simulink model "Simulacao"  (R2015a)
settings: Solver=ode45  StartTime=0.0  StopTime=25  RelTol=1e-3
undefined symbols (not defined in the file): K, Kd, Ki, Kp, T, teta
settings Model: Creator=Alunos  LastModifiedBy=Miguel Gameiro

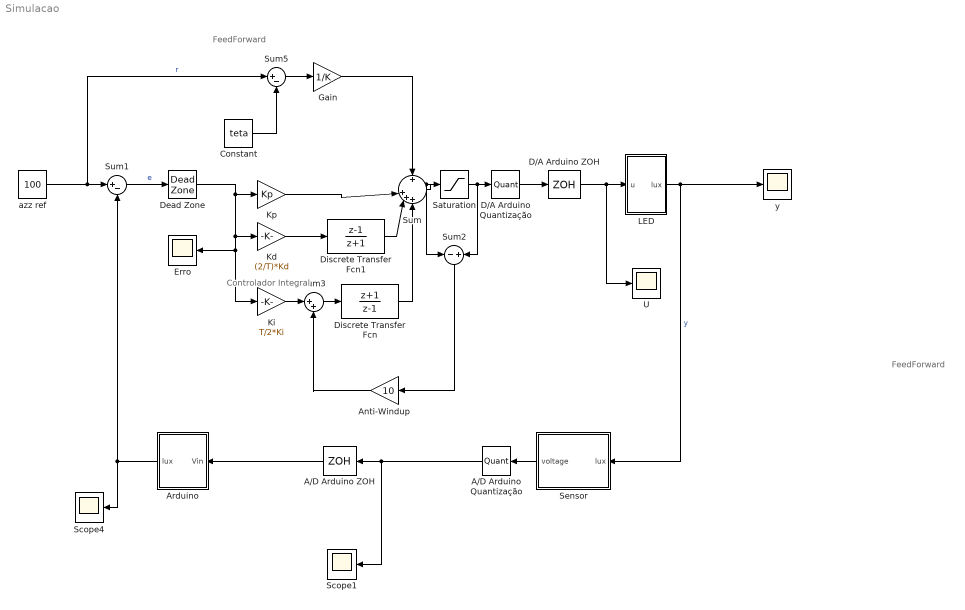
== system Simulacao ==
  note: Controlador Integral
  note: FeedForward
  note: FeedForward
  A/D Arduino Quantização : Quantizer  QuantizationInterval=5/1024
  A/D Arduino ZOH : ZeroOrderHold  SampleTime=T
  Anti-Windup : Gain  Gain=10
  Arduino : Subsystem
  Constant : Constant  Value=teta
  D/A Arduino ZOH : ZeroOrderHold  SampleTime=T
  D/A Arduino Quantização : Quantizer  QuantizationInterval=5/255
  Dead Zone : DeadZone  LowerValue=-6  UpperValue=6  SaturateOnIntegerOverflow=on
  Discrete Transfer Fcn : DiscreteTransferFcn  Numerator=[1 1]  Denominator=[1 -1]  SampleTime=T
  Discrete Transfer Fcn1 : DiscreteTransferFcn  Numerator=[1 -1]  Denominator=[1 1]  SampleTime=T
  Erro : Scope
      settings: SaveName=ScopeData2
  Gain : Gain  Gain=1/K
  Kd : Gain  Gain=(2/T)*Kd
  Ki : Gain  Gain=T/2*Ki
  Kp : Gain  Gain=Kp
  LED : Subsystem
  Saturation : Saturate  UpperLimit=5  LowerLimit=0
  Scope1 : Scope
  Scope4 : Scope
      settings: SaveName=ScopeData4
  Sensor : Subsystem
  Sum : Sum  Inputs=+||+++
  Sum1 : Sum  Inputs=|+-
  Sum2 : Sum  Inputs=-|+
  Sum3 : Sum  Inputs=|++
  Sum5 : Sum  Inputs=|+-
  U : Scope
      settings: SaveName=ScopeData3
  azz ref : Constant  Value=100
  y : Scope
      settings: SaveName=y
  wires:
  LED/1(lux) -> y/1, Sensor/1(lux)  "y"
  Saturation/1 -> Sum2/2, D/A Arduino Quantização/1
  Sensor/1(voltage) -> A/D Arduino Quantização/1
  azz ref/1 -> Sum5/1, Sum1/1  "r"
  Arduino/1(lux) -> Sum1/2, Scope4/1
  Sum1/1 -> Dead Zone/1  "e"
  D/A Arduino Quantização/1 -> D/A Arduino ZOH/1
  A/D Arduino Quantização/1 -> A/D Arduino ZOH/1, Scope1/1
  A/D Arduino ZOH/1 -> Arduino/1(Vin)
  Sum/1 -> Sum2/1, Saturation/1
  Kp/1 -> Sum/2
  D/A Arduino ZOH/1 -> U/1, LED/1(u)
  Dead Zone/1 -> Erro/1, Ki/1, Kd/1, Kp/1
  Ki/1 -> Sum3/1
  Sum3/1 -> Discrete Transfer Fcn/1
  Sum2/1 -> Anti-Windup/1
  Anti-Windup/1 -> Sum3/2
  Kd/1 -> Discrete Transfer Fcn1/1
  Discrete Transfer Fcn/1 -> Sum/4
  Discrete Transfer Fcn1/1 -> Sum/3
  Gain/1 -> Sum/1
  Sum5/1 -> Gain/1
  Constant/1 -> Sum5/2

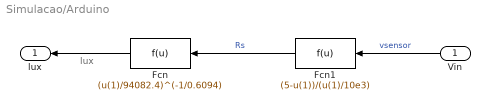
== system Simulacao/Arduino ==
  note: lux
  Vin : Inport
  Fcn : Fcn  Expr=(u(1)/94082.4)^(-1/0.6094)
  Fcn1 : Fcn  Expr=(5-u(1))/(u(1)/10e3)
  lux : Outport
  wires:
  Vin/1 -> Fcn1/1  "vsensor"
  Fcn/1 -> lux/1
  Fcn1/1 -> Fcn/1  "Rs"

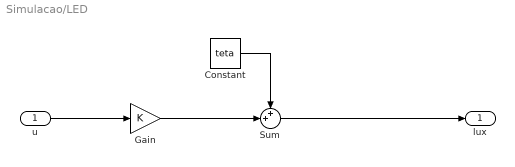
== system Simulacao/LED ==
  u : Inport
  Constant : Constant  Value=teta
  Gain : Gain  Gain=K
  Sum : Sum  Inputs=++|
  lux : Outport
  wires:
  Sum/1 -> lux/1
  Gain/1 -> Sum/2
  u/1 -> Gain/1
  Constant/1 -> Sum/1

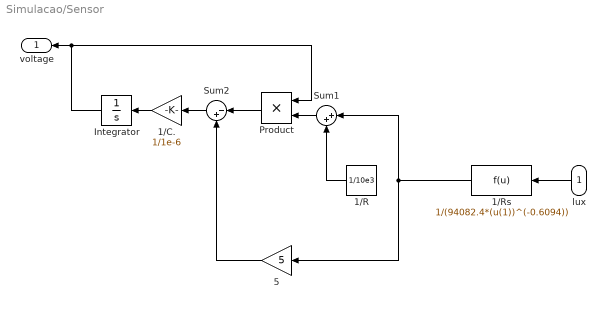
== system Simulacao/Sensor ==
  lux : Inport
  1/C. : Gain  Gain=1/1e-6
  1/R : Constant  Value=1/10e3
  1/Rs : Fcn  Expr=1/(94082.4*(u(1))^(-0.6094))
  5 : Gain  Gain=5
  Integrator : Integrator
  Product : Product
  Sum1 : Sum  Inputs=|++
  Sum2 : Sum  Inputs=|-+
  voltage : Outport
  wires:
  Integrator/1 -> Product/1, voltage/1
  Product/1 -> Sum2/1
  1/R/1 -> Sum1/2
  Sum2/1 -> 1/C./1
  1/Rs/1 -> 5/1, Sum1/1
  5/1 -> Sum2/2
  Sum1/1 -> Product/2
  lux/1 -> 1/Rs/1
  1/C./1 -> Integrator/1
